simulink model "BipolarCoding"  (R2024b)
settings: Solver=VariableStepAuto  StartTime=0.0  StopTime=16  RelTol=1e-3
libraries: commrandsrc3 x1, dspmathops x1
settings Model: Creator=gupta
settings RTWCC: GPUComputeCapability=3.5

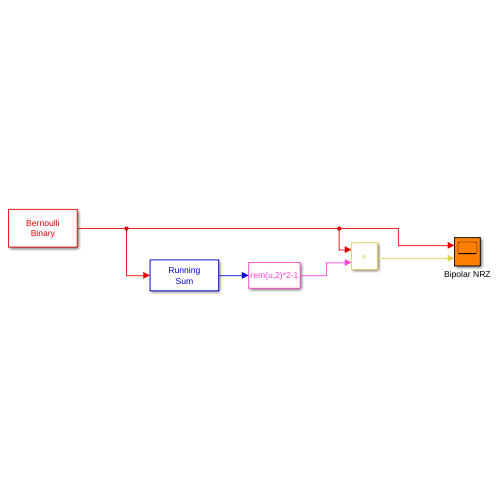
[thumbnail: Simulink's stored preview of the top-level diagram]
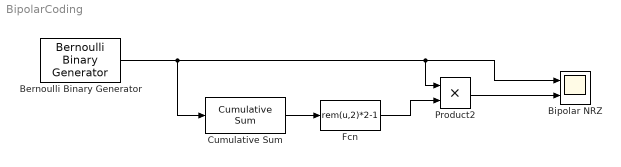
== system BipolarCoding ==
  Bernoulli Binary Generator : commrandsrc3/Bernoulli Binary Generator  ProbabilityOfZero=0.5  SeedSource=Auto  Seed=0  SampleTime=1  SamplesPerFrame=1  OutputDataType=double  SimulateUsing=Interpreted execution
  Bipolar NRZ : Scope  NumInputPorts=2
  Cumulative Sum : dspmathops/Cumulative Sum  dim=Channels (running sum)  InputProcessing=Columns as channels (frame based)  reset_popup=None  roundingMode=Floor  overflowMode=off  outputDataTypeStr=Inherit: Same as accumulator  outputMin=[]  outputMax=[]  outputLastDataTypeStr=Inherit: Same as accumulator
  Fcn : Fcn  Expr=rem(u,2)*2-1
  Product2 : Product
  wires:
  Bernoulli Binary Generator/1 -> Cumulative Sum/1, Product2/1, Bipolar NRZ/1
  Cumulative Sum/1 -> Fcn/1
  Product2/1 -> Bipolar NRZ/2
  Fcn/1 -> Product2/2
